simulink model "velocity_control_loop"  (R2015b)
settings: Solver=VariableStepAuto  StartTime=0.0  StopTime=50  RelTol=1e-3
PreLoadFcn:
  | boat_constants
values from neighbouring files (symbols this model uses):
  A = (Kt/(Ra*J))*(T)    (= 10277.8160138)    [boat_constants.m]
  B = (1/J)*(b + (Kt*Kb)/Ra)    (= 1910.04099303)    [boat_constants.m]
  m = 19.3    [boat_constants.m]
libraries: simulink x1
settings Model: Creator=NicolasFonteyne  LastModifiedBy=NicolasFonteyne

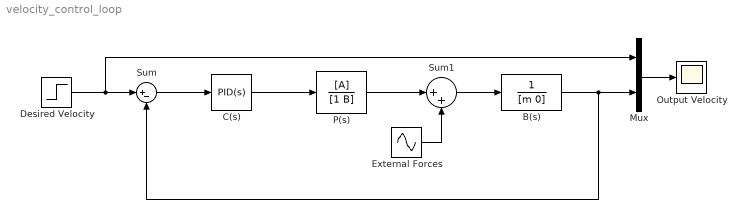
== system velocity_control_loop ==
  B(s) : TransferFcn  Denominator=[m 0]
  C(s) : simulink/Continuous/PID Controller  Controller=PID  TimeDomain=Continuous-time  SampleTime=-1  IntegratorMethod=Trapezoidal  FilterMethod=Forward Euler  Form=Parallel  UseFilter=off  ControllerParametersSource=internal  P=4.56054468973139  I=1.07387671482573  D=0.652167710532266  N=4.862432089028  InitialConditionSource=internal  InitialConditionForIntegrator=0  InitialConditionForFilter=0  ExternalReset=none  LimitOutput=on  UpperSaturationLimit=12  LowerSaturationLimit=-12  LinearizeAsGain=on  AntiWindupMode=none  Kb=1  TrackingMode=off  Kt=1  PParamMin=[]  PParamMax=[]  IParamMin=[]  IParamMax=[]  DParamMin=[]  DParamMax=[]  NParamMin=[]  NParamMax=[]  KbParamMin=[]  KbParamMax=[]  KtParamMin=[]  KtParamMax=[]  POutMin=[]  POutMax=[]  IOutMin=[]  IOutMax=[]  DOutMin=[]  DOutMax=[]  NOutMin=1000000  NOutMax=1000000000000000000000  KbOutMin=[]  KbOutMax=[]  KtOutMin=[]  KtOutMax=[]  IntegratorOutMin=[]  IntegratorOutMax=[]  FilterOutMin=[]  FilterOutMax=[]  SumOutMin=[]  SumOutMax=[]  SumI1OutMin=[]  SumI1OutMax=[]  SumI2OutMin=[]  SumI2OutMax=[]  SumI3OutMin=[]  SumI3OutMax=[]  SumDOutMin=[]  SumDOutMax=[]  SaturationOutMin=[]  SaturationOutMax=[]  IntegratorContinuousStateAttributes=''  IntegratorStateMustResolveToSignalObject=off  IntegratorRTWStateStorageClass=Auto  FilterContinuousStateAttributes=''  FilterStateMustResolveToSignalObject=off  FilterRTWStateStorageClass=Auto  DifferentiatorICPrevScaledInput=0  DifferentiatorOutMin=[]  DifferentiatorOutMax=[]
  "Desired Velocity\t" : Step  Time=0  SampleTime=0
  External Forces : Sin  Amplitude=.5  Frequency=.5  SampleTime=0
  Mux : Mux  Inputs=2
  Output Velocity : Scope
  P(s) : TransferFcn  Numerator=[A]  Denominator=[1 B]
  Sum : Sum  Inputs=|+-
  Sum1 : Sum  Inputs=|++
  wires:
  "Desired Velocity\t"/1 -> Mux/1, Sum/1
  Sum/1 -> C(s)/1
  B(s)/1 -> Sum/2, Mux/2
  Sum1/1 -> B(s)/1
  Mux/1 -> Output Velocity/1
  C(s)/1 -> P(s)/1
  External Forces/1 -> Sum1/2
  P(s)/1 -> Sum1/1
